simulink model "untitled"  (R2025b)
settings: Solver=VariableStepAuto  StartTime=0.0  StopTime=10.0  RelTol=1e-3
settings Model: Creator=Collin  LastModifiedBy=Collin

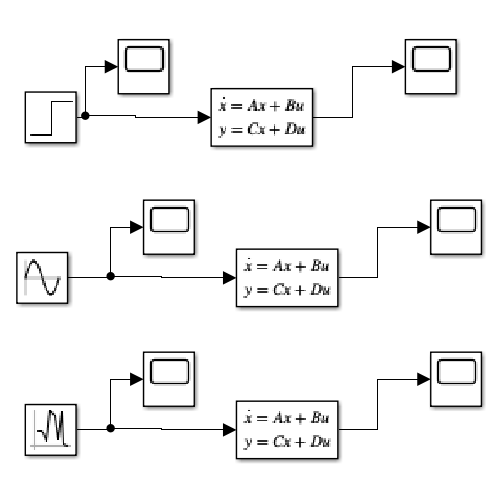
[thumbnail: Simulink's stored preview of the top-level diagram]
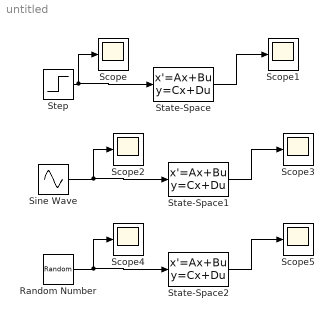
== system untitled ==
  Random Number : RandomNumber  SampleTime=0.1
  Scope{,1..5} (6 alike) : Scope
      Scope settings: ActiveDisplayYMinimum=-0.12499999999999997  ActiveDisplayYMaximum=1.125
      Scope1 settings: ActiveDisplayYMinimum=-17.205156895762574  ActiveDisplayYMaximum=54.846412061863184
      Scope2 settings: ActiveDisplayYMinimum=-1  ActiveDisplayYMaximum=1  DataLoggingVariableName=ScopeData2
      Scope3 settings: ActiveDisplayYMinimum=-31.705069480684834  ActiveDisplayYMaximum=74.747913309302419  DataLoggingVariableName=ScopeData3
      Scope4 settings: ActiveDisplayYMinimum=-3.0455098440395796  ActiveDisplayYMaximum=2.5811634537908086  DataLoggingVariableName=ScopeData4
      Scope5 settings: ActiveDisplayYMinimum=-17.205156895762574  ActiveDisplayYMaximum=54.846412061863184  DataLoggingVariableName=ScopeData5
  Sine Wave : Sin  SampleTime=0
  State-Space : StateSpace  A=|  B=[1; 0; -3; 6; 2;];  C=[2, -4, 0, 0, 9];  InitialCondition=[randi([0 10]), randi([0 10]), randi([0 10]), randi([0 10]), randi([0 10])]
      | [-8, 7, 0, -3, -5;
      | 0, -4, 0, 6, 8;
      | -3, 7, -3, -6, 5; 0, 0, 0, -5, 0; 0, 0, 0, 10, -1];
  State-Space1 : StateSpace  A=|  B=[1; 0; -3; 6; 2;];  C=[2, -4, 0, 0, 9];  D=0  InitialCondition=[randi([0 10]), randi([0 10]), randi([0 10]), randi([0 10]), randi([0 10])]
      | [-8, 7, 0, -3, -5;
      |         0, -4, 0, 6, 8;
      |         -3, 7, -3, -6, 5;
      |         0, 0, 0, -5, 0;
      |         0, 0, 0, 10, -1];
  State-Space2 : StateSpace  A=|  B=[1; 0; -3; 6; 2;];  C=[2, -4, 0, 0, 9];  D=0  InitialCondition=[randi([0 10]), randi([0 10]), randi([0 10]), randi([0 10]), randi([0 10])]
      | [-8, 7, 0, -3, -5;
      |         0, -4, 0, 6, 8;
      |         -3, 7, -3, -6, 5;
      |         0, 0, 0, -5, 0;
      |         0, 0, 0, 10, -1];
  Step : Step  SampleTime=0
  wires:
  Step/1 -> State-Space/1, Scope/1
  State-Space/1 -> Scope1/1
  State-Space1/1 -> Scope3/1
  Sine Wave/1 -> State-Space1/1, Scope2/1
  State-Space2/1 -> Scope5/1
  Random Number/1 -> State-Space2/1, Scope4/1
